simulink model "sim_model"  (Simulink 9.2)
settings: Solver=ode45  StartTime=0  StopTime=60  RelTol=0.001  EnableMultiTasking=on
libraries: fmu_me_lib x1
settings Model: Creator=Tin Rabuzin  LastModifiedBy=meagh
settings DataIOCC: SignalLoggingSaveFormat=Dataset  OutputSaveName=simout  OutputOption=SpecifiedOutputTimes  OutputTimes=[0:0.12:60]
settings OptimizationCC: ExpressionDepthLimit=2147483647
settings DebuggingCC: SolverPrmCheckMsg=warning

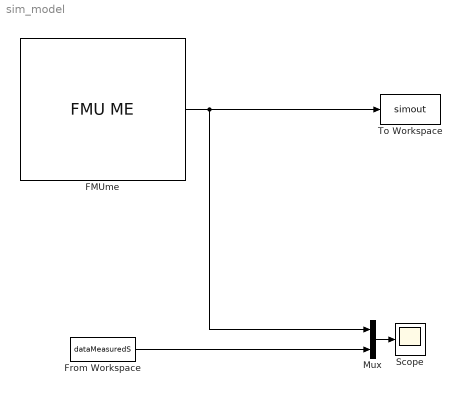
== system sim_model ==
  FMUme : fmu_me_lib/FMU ME  Description=Simulates an FMU for Model Exchange 1.0 or Model Exchange 2.0.  dummy=0
      settings: SourceProductName=The database C:\Users\meagh\AppData\Roaming\MathWorks\MATLAB\R2018b\slblocks_master.db is locked, or a table in the database is locked. (database is locked)
  From Workspace : FromWorkspace  VariableName=dataMeasuredS  SampleTime=0
  Mux : Mux  Inputs=2
  Scope : Scope
  To Workspace : ToWorkspace  VariableName=simout  SaveFormat=Structure With Time  SampleTime=-1
  wires:
  FMUme/1 -> Mux/1, To Workspace/1
  From Workspace/1 -> Mux/2
  Mux/1 -> Scope/1
